simulink model "modelNum"  (R2015a)
settings: Solver=ode45  StartTime=0.0  StopTime=10.0  RelTol=1e-3
undefined symbols (not defined in the file): sys
libraries: simulink x1
settings Model: Creator=user  LastModifiedBy=user

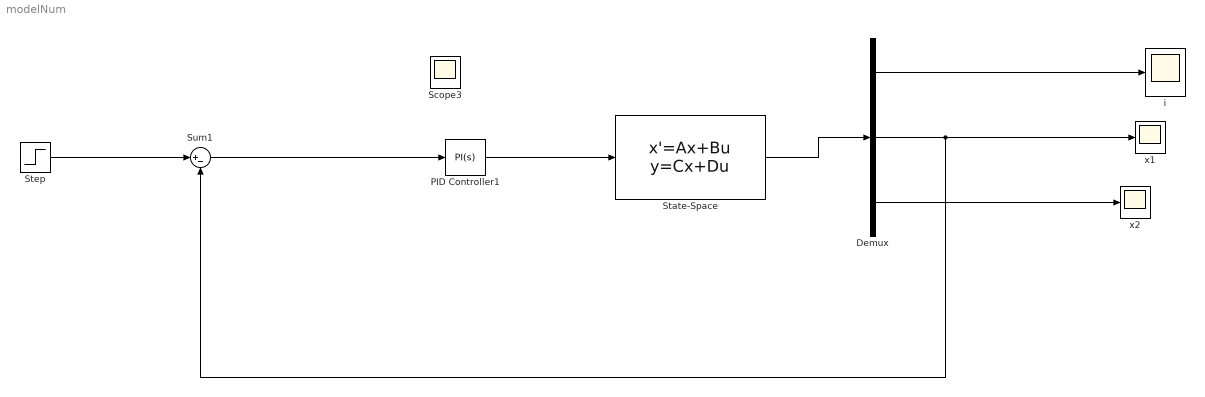
== system modelNum ==
  Demux : Demux  Outputs=3
  PID Controller1 : simulink/Continuous/PID Controller  Controller=PI  TimeDomain=Continuous-time  SampleTime=-1  IntegratorMethod=Forward Euler  FilterMethod=Forward Euler  Form=Parallel  UseFilter=on  ControllerParametersSource=internal  P=-0.159200719143865  I=-3.50493634442111  D=-1.07085550287524  N=22115.1807595506  InitialConditionSource=internal  InitialConditionForIntegrator=0  InitialConditionForFilter=0  ExternalReset=none  LimitOutput=off  UpperSaturationLimit=inf  LowerSaturationLimit=-inf  LinearizeAsGain=on  AntiWindupMode=none  Kb=1  TrackingMode=off  Kt=1  PParamMin=[]  PParamMax=[]  IParamMin=[]  IParamMax=[]  DParamMin=[]  DParamMax=[]  NParamMin=[]  NParamMax=[]  KbParamMin=[]  KbParamMax=[]  KtParamMin=[]  KtParamMax=[]  POutMin=[]  POutMax=[]  IOutMin=[]  IOutMax=[]  DOutMin=[]  DOutMax=[]  NOutMin=[]  NOutMax=[]  KbOutMin=[]  KbOutMax=[]  KtOutMin=[]  KtOutMax=[]  IntegratorOutMin=[]  IntegratorOutMax=[]  FilterOutMin=[]  FilterOutMax=[]  SumOutMin=[]  SumOutMax=[]  SumI1OutMin=[]  SumI1OutMax=[]  SumI2OutMin=[]  SumI2OutMax=[]  SumI3OutMin=[]  SumI3OutMax=[]  SumDOutMin=[]  SumDOutMax=[]  SaturationOutMin=[]  SaturationOutMax=[]  IntegratorContinuousStateAttributes=''  IntegratorStateMustResolveToSignalObject=off  IntegratorRTWStateStorageClass=Auto  FilterContinuousStateAttributes=''  FilterStateMustResolveToSignalObject=off  FilterRTWStateStorageClass=Auto  DifferentiatorICPrevScaledInput=0  DifferentiatorOutMin=[]  DifferentiatorOutMax=[]
  Scope3 : Scope
      settings: TimeRange=2.475095785440614  YMin=3885000.000000001  YMax=8411666.666666668  SaveName=ScopeData4
  State-Space : StateSpace  A=sys.a  B=sys.b  C=sys.c  D=sys.d  X0=0
  Step : Step  SampleTime=0
  Sum1 : Sum  Inputs=|+-
  i : Scope
      settings: YMin=-0.25393  YMax=2.28535
  x1 : Scope
      settings: TimeRange=10  YMin=-10  YMax=15  SaveName=ScopeData2
  x2 : Scope
      settings: TimeRange=10  YMin=-10  YMax=15  SaveName=ScopeData3
  wires:
  Demux/1 -> i/1
  State-Space/1 -> Demux/1
  Demux/2 -> Sum1/2, x1/1
  Demux/3 -> x2/1
  Sum1/1 -> PID Controller1/1
  PID Controller1/1 -> State-Space/1
  Step/1 -> Sum1/1
